simulink model "deadbeat"  (R2018a)
settings: Solver=VariableStepAuto  StartTime=0.0  StopTime=10.0  RelTol=1e-3
settings Model: Creator=GRENTOR  LastModifiedBy=GRENTOR

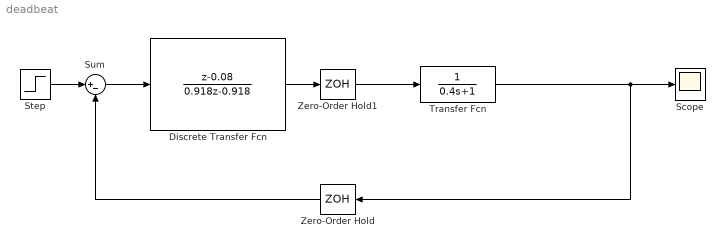
== system deadbeat ==
  Discrete Transfer Fcn : DiscreteTransferFcn  Numerator=[1 -0.08]  Denominator="[0.918  -0.918 ]"  SampleTime=1
  Scope : Scope
  Step : Step  SampleTime=1
  Sum : Sum  Inputs=|+-
  Transfer Fcn : TransferFcn  Denominator=[0.4 1]
  Zero-Order Hold : ZeroOrderHold
  Zero-Order Hold1 : ZeroOrderHold
  wires:
  Zero-Order Hold/1 -> Sum/2
  Step/1 -> Sum/1
  Sum/1 -> Discrete Transfer Fcn/1
  Discrete Transfer Fcn/1 -> Zero-Order Hold1/1
  Zero-Order Hold1/1 -> Transfer Fcn/1
  Transfer Fcn/1 -> Zero-Order Hold/1, Scope/1
